simulink model "ukol_1_a_bez_sumu"  (R2017a)
settings: Solver=VariableStepAuto  StartTime=0.0  StopTime=100  MaxStep=1e-1  RelTol=1e-3  EnableMultiTasking=on
libraries: cstblocks x1
settings Model: Creator=kuhaj  LastModifiedBy=tomas
settings DataIOCC: LimitDataPoints=on
settings OptimizationCC: LifeSpan=inf
settings DebuggingCC: AllowSymbolicDim=off  SFUnexpectedBacktrackingDiag=warning  SFNoUnconditionalDefaultTransitionDiag=warning  SFExecutionAtInitializationDiag=none
settings ModelReferenceCC: PropagateSignalLabelsOutOfModel=off
settings GRTTargetCC: TargetLangStandard=C89/C90 (ANSI)
settings ConfigComp: CovMetricSettings=dw  CovHtmlReporting=on  CovSaveCumulativeToWorkspaceVar=on  CovSaveSingleToWorkspaceVar=on  CovExternalEMLEnable=off

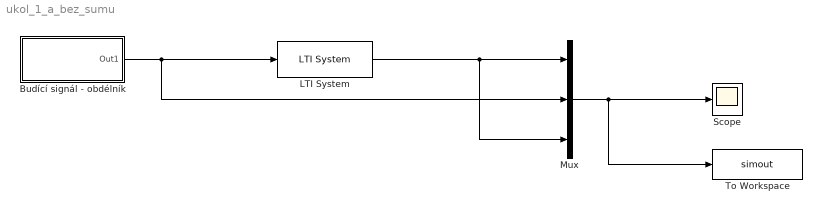
== system ukol_1_a_bez_sumu ==
  Budící signál - obdélník : Subsystem
  LTI System : cstblocks/LTI System  sys=discrete_Fs  IC=[]
  Mux : Mux  Inputs=3
  Scope : Scope
  To Workspace : ToWorkspace  VariableName=simout  SaveFormat=Timeseries  SampleTime=-1
  wires:
  Mux/1 -> To Workspace/1, Scope/1
  LTI System/1 -> Mux/3, Mux/1
  Budící signál - obdélník/1(Out1) -> LTI System/1, Mux/2

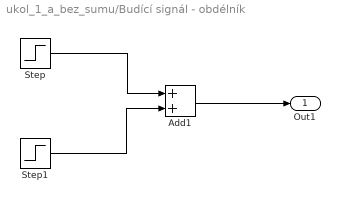
== system ukol_1_a_bez_sumu/Budící signál - obdélník ==
  Add1 : Sum
  Step : Step  SampleTime=0
  Step1 : Step  Time=2  After=-1  SampleTime=0
  Out1 : Outport
  wires:
  Step1/1 -> Add1/2
  Step/1 -> Add1/1
  Add1/1 -> Out1/1
